simulink model "deadbeat_smm_with_lqr"  (R2015a)
settings: Solver=FixedStepDiscrete  SolverMode=SingleTasking  StartTime=0.0  StopTime=inf  FixedStep=sample_time  RelTol=1e-3
undefined symbols (not defined in the file or in its folder): A_kalman_fourbar_gear, A_kalman_transverse, A_kalman_vertical, A_lpf_accelerometer, A_lpf_fourbar_angles, A_lpf_imu, A_lpf_lateral_angle, B1_lpf_accelerometer, B1_lpf_fourbar_angles, B1_lpf_imu, B1_lpf_lateral_angle, B2_lpf_accelerometer, B2_lpf_fourbar_angles, B2_lpf_imu, B2_lpf_lateral_angle, B_dx_versus_x0, B_kalman_fourbar_gear, B_kalman_transverse, B_kalman_vertical, backwards_K_sag_of_t, backwards_P_sag_of_t, C_kalman_fourbar_gear, C_kalman_transverse, C_kalman_vertical, com_leg_motor, com_torso, contact_threshold, control_start_time, d_ankle_to_foot, d_vertical_com, desired_com_forward_velocity, desired_com_lateral_velocity, desired_initial_leg_roll_left, desired_initial_leg_roll_right, desired_stance_beta2, desired_standing_torso_pitch, desired_standing_torso_roll, desired_standing_z, desired_torso_pitch, desired_torso_roll, Discrete, enable_bouncing, fcut_contact, fdesignblkfcn, forward_dx_of_dxstar, forward_x_of_dxstar, g, gcbh, HIP_MTR_MAX_CONT_TORQUE, HIP_MTR_MAX_TORQUE, i_leg_motor, i_robot, i_torso, initial_dx_estimate, initial_dy_estimate, initial_dz_estimate, initial_leg_selection, initial_z_estimate, k_lateral_accel_for_torso_roll, k_lateral_swing_on_boom ... (+77)
libraries: simulink x21, ctrlSharedLib x7, dsparch4 x3
(part 3 of 5)

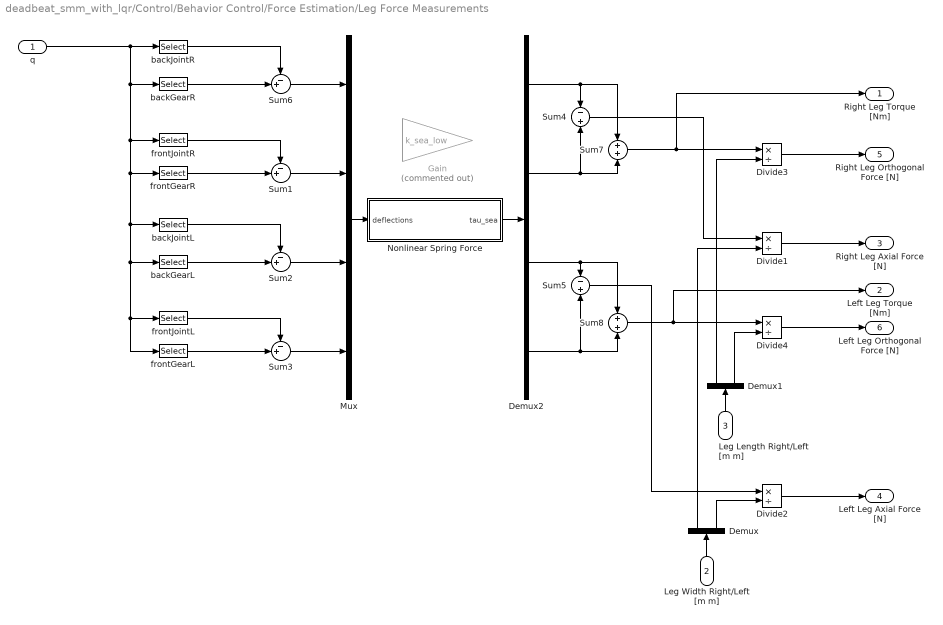
== system deadbeat_smm_with_lqr/Control/Behavior Control/Force Estimation/Leg Force Measurements ==
  q : Inport
  Leg Width Right/Left [m m] : Inport  Port=2
  Leg Length Right/Left [m m] : Inport  Port=3
  Demux : Demux  Outputs=2
  Demux1 : Demux  Outputs=2
  Demux2 : Demux
  Divide{1..4} (4 alike) : Product  Inputs=*/
  Gain : Gain  Commented=on  Gain=k_sea_low
  Mux : Mux
  Nonlinear Spring Force : MATLAB Function  TreatAsAtomicUnit=on
  Sum{1..3,6} (4 alike) : Sum  Inputs=-+|
  Sum4 : Sum  Inputs=-|+
  Sum5 : Sum  Inputs=-|+
  Sum7 : Sum  Inputs=+|+
  Sum8 : Sum  Inputs=+|+
  backGearL : Selector  InputPortWidth=13  Indices=[6]
  backGearR : Selector  InputPortWidth=13  Indices=[2]
  backJointL : Selector  InputPortWidth=13  Indices=[5]
  backJointR : Selector  InputPortWidth=13  Indices=[1]
  frontGearL : Selector  InputPortWidth=13  Indices=[8]
  frontGearR : Selector  InputPortWidth=13  Indices=[4]
  frontJointL : Selector  InputPortWidth=13  Indices=[7]
  frontJointR : Selector  InputPortWidth=13  Indices=[3]
  Right Leg Torque [Nm] : Outport
  Left Leg Torque [Nm] : Outport  Port=2
  Right Leg Axial Force [N] : Outport  Port=3
  Left Leg Axial Force [N] : Outport  Port=4
  Right Leg Orthogonal Force [N] : Outport  Port=5
  Left Leg Orthogonal Force [N] : Outport  Port=6
  wires:
  Nonlinear Spring Force/1(tau_sea) -> Demux2/1
  Mux/1 -> Nonlinear Spring Force/1(deflections)
  Divide4/1 -> Left Leg Orthogonal Force [N]/1
  Divide3/1 -> Right Leg Orthogonal Force [N]/1
  Leg Length Right/Left [m m]/1 -> Demux1/1
  Demux1/2 -> Divide4/2
  Demux1/1 -> Divide3/2
  Sum8/1 -> Left Leg Torque [Nm]/1, Divide4/1
  Sum7/1 -> Right Leg Torque [Nm]/1, Divide3/1
  Demux2/3 -> Sum5/1, Sum8/1
  Divide2/1 -> Left Leg Axial Force [N]/1
  Divide1/1 -> Right Leg Axial Force [N]/1
  Demux/2 -> Divide2/2
  Demux/1 -> Divide1/2
  Leg Width Right/Left [m m]/1 -> Demux/1
  Sum5/1 -> Divide2/1
  Sum4/1 -> Divide1/1
  Demux2/4 -> Sum8/2, Sum5/2
  Demux2/2 -> Sum4/2, Sum7/2
  Demux2/1 -> Sum7/1, Sum4/1
  q/1 -> backJointR/1, frontJointR/1, frontGearR/1, backGearL/1, frontGearL/1, frontJointL/1, backJointL/1, backGearR/1
  backGearR/1 -> Sum6/2
  frontJointR/1 -> Sum1/1
  frontGearR/1 -> Sum1/2
  backJointR/1 -> Sum6/1
  Sum1/1 -> Mux/2
  Sum6/1 -> Mux/1
  backGearL/1 -> Sum2/2
  frontJointL/1 -> Sum3/1
  frontGearL/1 -> Sum3/2
  backJointL/1 -> Sum2/1
  Sum2/1 -> Mux/3
  Sum3/1 -> Mux/4

== system deadbeat_smm_with_lqr/Control/Behavior Control/Force Estimation/Leg Plane GRF ==
  Axial Force [N] : Inport
  Orthogonal Force [N] : Inport  Port=2
  Torso Pitch [rad] : Inport  Port=3
  Leg Angle [rad] : Inport  Port=4
  Gain : Gain  Gain=-1
  Product : Product
  Product1 : Product
  Sum : Sum  Inputs=++|
  Sum1 : Sum  Inputs=+|+
  Trigonometric Function : Trigonometry  Operator=cos
  Trigonometric Function1 : Trigonometry
  Vertical Force [N] : Outport
  wires:
  Gain/1 -> Sum1/1
  Sum/1 -> Trigonometric Function1/1, Trigonometric Function/1
  Product/1 -> Gain/1
  Trigonometric Function/1 -> Product/2
  Torso Pitch [rad]/1 -> Sum/1
  Leg Angle [rad]/1 -> Sum/2
  Axial Force [N]/1 -> Product/1
  Orthogonal Force [N]/1 -> Product1/1
  Trigonometric Function1/1 -> Product1/2
  Sum1/1 -> Vertical Force [N]/1
  Product1/1 -> Sum1/2

== system deadbeat_smm_with_lqr/Control/Behavior Control/Primary and Lateral Behavior/Circular Buffer ==
  Flight [1/0] : Inport
  Exiting Stance [1/0] : Inport  Port=2
  Hopping [1/0] : Inport  Port=3
  dX [m/s] : Inport  Port=4
  dY [m/s] : Inport  Port=5
  X Foot Correction [m] : Inport  Port=6
  Y Foot Correction [m] : Inport  Port=7
  target dX [m/s] : Inport  Port=8
  target dY [m/s] : Inport  Port=9
  Buffer : MATLAB Function  TreatAsAtomicUnit=on  SystemSampleTime=sample_time
  Buffer1 : MATLAB Function  TreatAsAtomicUnit=on  SystemSampleTime=sample_time
  Buffer2 : MATLAB Function  TreatAsAtomicUnit=on  SystemSampleTime=sample_time
  Buffer3 : MATLAB Function  TreatAsAtomicUnit=on  SystemSampleTime=sample_time
  Buffer4 : MATLAB Function  TreatAsAtomicUnit=on  SystemSampleTime=sample_time
  Buffer5 : MATLAB Function  TreatAsAtomicUnit=on  SystemSampleTime=sample_time
  Buffer6 : MATLAB Function  TreatAsAtomicUnit=on  SystemSampleTime=sample_time
  Buffer7 : MATLAB Function  TreatAsAtomicUnit=on  SystemSampleTime=sample_time
  Demux : Demux  Outputs=6
  Detect Decrease : simulink/Logic and Bit Operations/Detect Decrease  vinit=0.0  InputProcessing=Inherited  OutDataTypeStr=boolean
  Enabled on Touchdown : Subsystem  TreatAsAtomicUnit=on
  Logical Operator : Logic  AllPortsSameDT=off  OutDataTypeStr=boolean
  Mux : Mux  Inputs=6
  buffer size5 : Constant  Value=recorded_steps
  "dX Touchdown History " : Outport
  X Foot Correction History : Outport  Port=2
  dX Takeoff History : Outport  Port=3
  "dY Touchdown History " : Outport  Port=4
  Y Foot Correction History : Outport  Port=5
  dY Takeoff History : Outport  Port=6
  target dX History : Outport  Port=7
  target dY History : Outport  Port=8
  wires:
  Buffer/1(buffer) -> "dX Touchdown History "/1
  Detect Decrease/1 -> Enabled on Touchdown/Enable
  Buffer1/1(buffer) -> X Foot Correction History/1
  Buffer2/1(buffer) -> dX Takeoff History/1
  Demux/1 -> Buffer/1(data)
  Demux/3 -> Buffer1/1(data)
  X Foot Correction [m]/1 -> Mux/3
  Buffer3/1(buffer) -> "dY Touchdown History "/1
  Buffer4/1(buffer) -> Y Foot Correction History/1
  Demux/2 -> Buffer3/1(data)
  Buffer5/1(buffer) -> dY Takeoff History/1
  Y Foot Correction [m]/1 -> Mux/4
  Demux/4 -> Buffer4/1(data)
  target dX [m/s]/1 -> Mux/5
  Buffer6/1(buffer) -> target dX History/1
  Buffer7/1(buffer) -> target dY History/1
  buffer size5/1 -> Buffer2/3(buffer_size), Buffer/3(buffer_size), Buffer7/3(buffer_size), Buffer6/3(buffer_size), Buffer4/3(buffer_size), Buffer1/3(buffer_size), Buffer3/3(buffer_size), Buffer5/3(buffer_size)
  Demux/6 -> Buffer7/1(data)
  Demux/5 -> Buffer6/1(data)
  target dY [m/s]/1 -> Mux/6
  Exiting Stance [1/0]/1 -> Buffer/2(trigger), Buffer7/2(trigger), Buffer6/2(trigger), Buffer4/2(trigger), Buffer1/2(trigger), Buffer3/2(trigger), Buffer2/2(trigger), Buffer5/2(trigger)
  Hopping [1/0]/1 -> Logical Operator/1
  dY [m/s]/1 -> Buffer5/1(data), Mux/2
  dX [m/s]/1 -> Buffer2/1(data), Mux/1
  Flight [1/0]/1 -> Logical Operator/2
  Logical Operator/1 -> Detect Decrease/1
  Mux/1 -> Enabled on Touchdown/1(In)
  Enabled on Touchdown/1(Out) -> Demux/1

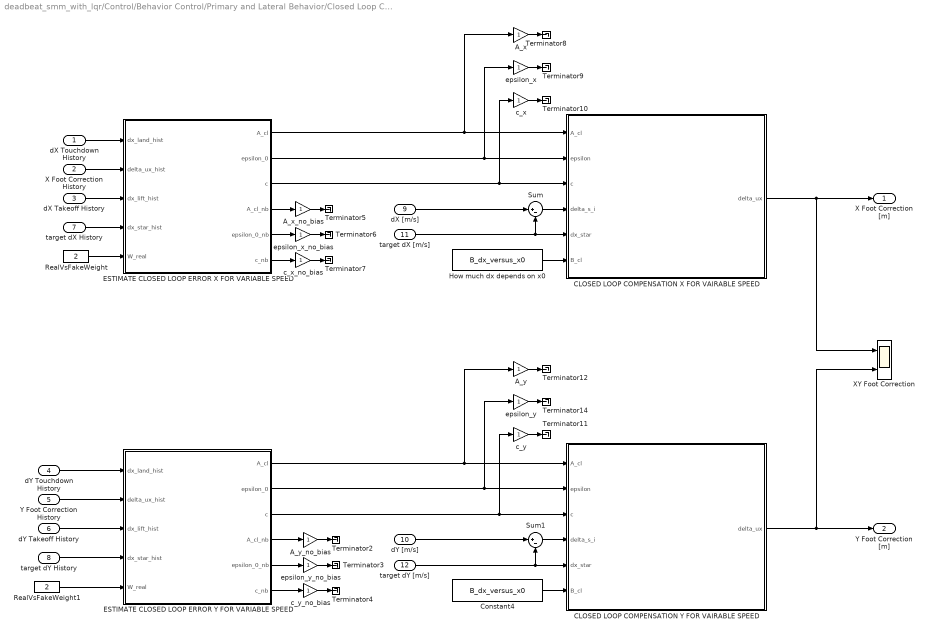
== system deadbeat_smm_with_lqr/Control/Behavior Control/Primary and Lateral Behavior/Closed Loop Compensation ==
  dX Touchdown History : Inport
  X Foot Correction History : Inport  Port=2
  dX Takeoff History : Inport  Port=3
  dY Touchdown History : Inport  Port=4
  Y Foot Correction History : Inport  Port=5
  dY Takeoff History : Inport  Port=6
  target dX History : Inport  Port=7
  target dY History : Inport  Port=8
  dX [m/s] : Inport  Port=9
  dY [m/s] : Inport  Port=10
  target dX [m/s] : Inport  Port=11
  "target dY [m/s] " : Inport  Port=12
  A_x : Gain
  A_x_no_bias : Gain
  A_y : Gain
  A_y_no_bias : Gain
  CLOSED LOOP COMPENSATION X FOR VAIRABLE SPEED : MATLAB Function  TreatAsAtomicUnit=on
  CLOSED LOOP COMPENSATION Y FOR VAIRABLE SPEED : MATLAB Function  TreatAsAtomicUnit=on
  Constant4 : Constant  Value=B_dx_versus_x0
  ESTIMATE CLOSED LOOP ERROR X FOR VARIABLE SPEED : MATLAB Function  TreatAsAtomicUnit=on
  ESTIMATE CLOSED LOOP ERROR Y FOR VARIABLE SPEED : MATLAB Function  TreatAsAtomicUnit=on
  How much dx depends on x0 : Constant  Value=B_dx_versus_x0
  RealVsFakeWeight : Constant  Value=2
  RealVsFakeWeight1 : Constant  Value=2
  Sum : Sum  Inputs=|+-
  Sum1 : Sum  Inputs=|+-
  Terminator{2..12,14} (12 alike) : Terminator
  XY Foot Correction : Scope  NumInputPorts=2
      settings: YMin=-1~-0.8  YMax=1~1.4  SaveName=ScopeData39  SampleInput=on
  c_x : Gain
  c_x_no_bias : Gain
  c_y : Gain
  c_y_no_bias : Gain
  epsilon_x : Gain
  epsilon_x_no_bias : Gain
  epsilon_y : Gain
  epsilon_y_no_bias : Gain
  X Foot Correction [m] : Outport
  Y Foot Correction [m] : Outport  Port=2
  wires:
  c_y/1 -> Terminator11/1
  epsilon_y/1 -> Terminator14/1
  A_y/1 -> Terminator12/1
  ESTIMATE CLOSED LOOP ERROR Y FOR VARIABLE SPEED/1(A_cl) -> CLOSED LOOP COMPENSATION Y FOR VAIRABLE SPEED/1(A_cl), A_y/1
  ESTIMATE CLOSED LOOP ERROR Y FOR VARIABLE SPEED/2(epsilon_0) -> CLOSED LOOP COMPENSATION Y FOR VAIRABLE SPEED/2(epsilon), epsilon_y/1
  ESTIMATE CLOSED LOOP ERROR Y FOR VARIABLE SPEED/3(c) -> CLOSED LOOP COMPENSATION Y FOR VAIRABLE SPEED/3(c), c_y/1
  c_x/1 -> Terminator10/1
  epsilon_x/1 -> Terminator9/1
  A_x/1 -> Terminator8/1
  ESTIMATE CLOSED LOOP ERROR X FOR VARIABLE SPEED/1(A_cl) -> CLOSED LOOP COMPENSATION X FOR VAIRABLE SPEED/1(A_cl), A_x/1
  ESTIMATE CLOSED LOOP ERROR X FOR VARIABLE SPEED/2(epsilon_0) -> CLOSED LOOP COMPENSATION X FOR VAIRABLE SPEED/2(epsilon), epsilon_x/1
  ESTIMATE CLOSED LOOP ERROR X FOR VARIABLE SPEED/3(c) -> CLOSED LOOP COMPENSATION X FOR VAIRABLE SPEED/3(c), c_x/1
  ESTIMATE CLOSED LOOP ERROR Y FOR VARIABLE SPEED/6(c_nb) -> c_y_no_bias/1
  ESTIMATE CLOSED LOOP ERROR Y FOR VARIABLE SPEED/5(epsilon_0_nb) -> epsilon_y_no_bias/1
  ESTIMATE CLOSED LOOP ERROR Y FOR VARIABLE SPEED/4(A_cl_nb) -> A_y_no_bias/1
  c_y_no_bias/1 -> Terminator4/1
  epsilon_y_no_bias/1 -> Terminator3/1
  A_y_no_bias/1 -> Terminator2/1
  c_x_no_bias/1 -> Terminator7/1
  epsilon_x_no_bias/1 -> Terminator6/1
  A_x_no_bias/1 -> Terminator5/1
  ESTIMATE CLOSED LOOP ERROR X FOR VARIABLE SPEED/4(A_cl_nb) -> A_x_no_bias/1
  ESTIMATE CLOSED LOOP ERROR X FOR VARIABLE SPEED/5(epsilon_0_nb) -> epsilon_x_no_bias/1
  ESTIMATE CLOSED LOOP ERROR X FOR VARIABLE SPEED/6(c_nb) -> c_x_no_bias/1
  CLOSED LOOP COMPENSATION Y FOR VAIRABLE SPEED/1(delta_ux) -> Y Foot Correction [m]/1, XY Foot Correction/2
  CLOSED LOOP COMPENSATION X FOR VAIRABLE SPEED/1(delta_ux) -> X Foot Correction [m]/1, XY Foot Correction/1
  Sum1/1 -> CLOSED LOOP COMPENSATION Y FOR VAIRABLE SPEED/4(delta_s_i)
  dY Touchdown History/1 -> ESTIMATE CLOSED LOOP ERROR Y FOR VARIABLE SPEED/1(dx_land_hist)
  dX [m/s]/1 -> Sum/1
  dX Touchdown History/1 -> ESTIMATE CLOSED LOOP ERROR X FOR VARIABLE SPEED/1(dx_land_hist)
  dX Takeoff History/1 -> ESTIMATE CLOSED LOOP ERROR X FOR VARIABLE SPEED/3(dx_lift_hist)
  X Foot Correction History/1 -> ESTIMATE CLOSED LOOP ERROR X FOR VARIABLE SPEED/2(delta_ux_hist)
  target dX History/1 -> ESTIMATE CLOSED LOOP ERROR X FOR VARIABLE SPEED/4(dx_star_hist)
  target dX [m/s]/1 -> CLOSED LOOP COMPENSATION X FOR VAIRABLE SPEED/5(dx_star), Sum/2
  Sum/1 -> CLOSED LOOP COMPENSATION X FOR VAIRABLE SPEED/4(delta_s_i)
  How much dx depends on x0/1 -> CLOSED LOOP COMPENSATION X FOR VAIRABLE SPEED/6(B_cl)
  RealVsFakeWeight/1 -> ESTIMATE CLOSED LOOP ERROR X FOR VARIABLE SPEED/5(W_real)
  dY [m/s]/1 -> Sum1/1
  dY Takeoff History/1 -> ESTIMATE CLOSED LOOP ERROR Y FOR VARIABLE SPEED/3(dx_lift_hist)
  Y Foot Correction History/1 -> ESTIMATE CLOSED LOOP ERROR Y FOR VARIABLE SPEED/2(delta_ux_hist)
  target dY History/1 -> ESTIMATE CLOSED LOOP ERROR Y FOR VARIABLE SPEED/4(dx_star_hist)
  "target dY [m/s] "/1 -> CLOSED LOOP COMPENSATION Y FOR VAIRABLE SPEED/5(dx_star), Sum1/2
  Constant4/1 -> CLOSED LOOP COMPENSATION Y FOR VAIRABLE SPEED/6(B_cl)
  RealVsFakeWeight1/1 -> ESTIMATE CLOSED LOOP ERROR Y FOR VARIABLE SPEED/5(W_real)

== system deadbeat_smm_with_lqr/Control/Behavior Control/Primary and Lateral Behavior/Enabled on Takeoff ==
  In : Inport
  Enable : EnablePort
  Out : Outport
  wires:
  In/1 -> Out/1

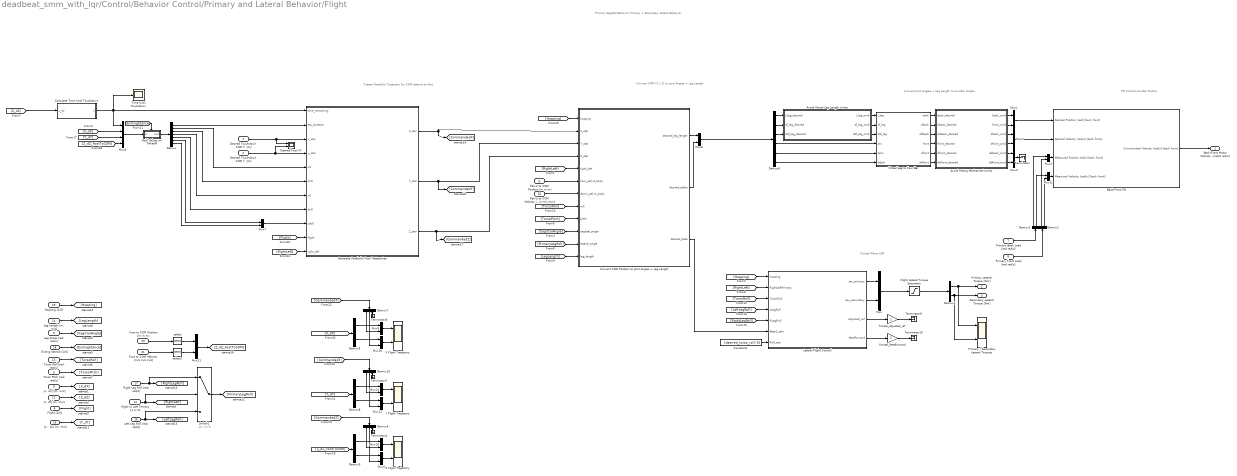
== system deadbeat_smm_with_lqr/Control/Behavior Control/Primary and Lateral Behavior/Flight ==
  note: Frontal Plane LQR
  note: PD Control Fourbar Motors
  note: Convert Joint Angles + Leg Length
      | to Fourbar Angles
  note: Convert COM (X,Y,Z) to
      | Joint Angles + Leg Length
  note: Create Parabolic
      | Trajectory for COM relative to foot
  note: Primary Sagittal Behavior
      | Primary + Secondary Lateral Behavior
  Desired Touchdown COM X  [m] : Inport
  Desired Touchdown COM Y  [m] : Inport  Port=2
  Torso Pitch [rad rad/s] : Inport  Port=3
  Flight [1/0] : Inport  Port=4
  Leg Angle [rad rad/s] : Inport  Port=5
  "[x, dx] [m, m/s]" : Inport  Port=6
  Primary Back Load [rad rad/s] : Inport  Port=7
  Primary Front Load [rad rad/s] : Inport  Port=8
  Pelvis to COM Position [m m m] : Inport  Port=9
  Pelvis to COM Velocity [m/s m/s m/s] : Inport  Port=10
  "[z, dz] [m, m/s]" : Inport  Port=11
  Right or Left Primary [1 or 0] : Inport  Port=12
  Torso Roll [rad rad/s] : Inport  Port=13
  "Leg Length [m, m/s]" : Inport  Port=14
  "[y,  dy] [m, m/s]" : Inport  Port=15
  "Left Leg Roll [rad, rad/s]" : Inport  Port=16
  "Right Leg Roll [rad, rad/s]" : Inport  Port=17
  Exiting Stance [1/0] : Inport  Port=18
  Hopping [1/0] : Inport  Port=19
  Foot to COM Position [m m m] : Inport  Port=20
  Foot to COM Velocity [m/s m/s m/s] : Inport  Port=21
  Avoid Hitting Mechanical Limits : MATLAB Function  TreatAsAtomicUnit=on
  Avoid Virtual Leg Length Limits : MATLAB Function  TreatAsAtomicUnit=on
  Back/Front PD : Subsystem
  Calculate Time Until Touchdown : MATLAB Function  TreatAsAtomicUnit=on
  Constant1 : Constant  Value=[desired_torso_roll; 0]
  "Convert COM Position to Joint Angles + Leg Length " : MATLAB Function  TreatAsAtomicUnit=on
  Demux : Demux  Outputs=7
  Demux{1..3,5,8..9} (6 alike) : Demux  Outputs=2
  Demux10 : Demux  Outputs=3
  Demux4 : Demux  Outputs=3
  Demux6 : Demux  Outputs=6
  Demux7 : Demux  Outputs=3
  Desired Foot XY : Scope  NumInputPorts=2
      settings: YMin=-1~-0.8  YMax=1~1.4  SaveName=ScopeData38  SampleInput=on
  Flight Lateral Torque Saturation : Saturate  UpperLimit=HIP_MTR_MAX_CONT_TORQUE  LowerLimit=-HIP_MTR_MAX_CONT_TORQUE
      settings: AttributesFormatString=Top: %<UpperLimit>\nBottom: %<LowerLimit>
  Generate Parabolic Foot Trajectories : MATLAB Function  TreatAsAtomicUnit=on
  Hold Values on Takeoff : Subsystem
  Lateral Flight Control : MATLAB Function  TreatAsAtomicUnit=on
  Mux{,1..5,7..13,15,21} (15 alike) : Mux  Inputs=2
  Mux6 : Mux
  Primary / Secondary Lateral Torques : Scope  NumInputPorts=2
      settings: YMin=-1~-0.8  YMax=1~1.4  SaveName=ScopeData32  SampleInput=on
  Switch1 : Switch  Criteria=u2 ~= 0
  Terminator{,4,6..7,9..10} (6 alike) : Terminator
  Time Until Touchdown : Scope
      settings: YMin=-1  YMax=1  SaveName=ScopeData37  SampleInput=on
  Virtual Leg to Four Bar : MATLAB Function  TreatAsAtomicUnit=on
  X Flight Trajectory : Scope  NumInputPorts=2
      settings: YMin=-1~-0.8  YMax=1~1.4  SaveName=ScopeData3  SampleInput=on
  Y Flight Trajectory : Scope  NumInputPorts=2
      settings: YMin=-1~-0.8  YMax=1~1.4  SaveName=ScopeData4  SampleInput=on
  Z Flight Trajectory : Scope  NumInputPorts=2
      settings: YMin=-1~-0.8  YMax=1~1.4  SaveName=ScopeData7  SampleInput=on
  frontal_adjusted_ref : Gain
  frontal_feedforward : Gain
  select : Selector  InputPortWidth=3  Indices=[3]
  select1 : Selector  InputPortWidth=3  Indices=[3]
  Back/Front Motor Velocity [rad/s rad/s] : Outport
  Primary Lateral Torque [Nm] : Outport  Port=2
  Secondary Lateral Torque [Nm] : Outport  Port=3
  wires:
  Mux3/1 -> Terminator/1
  Generate Parabolic Foot Trajectories/3(Z_star) -> [CommandedZ], "Convert COM Position to Joint Angles + Leg Length "/4(Z_star)
  [CommandedZ] -> Demux4/1
  [CommandedY] -> Demux10/1
  [CommandedX] -> Demux7/1
  Demux10/3 -> Terminator7/1
  [Y_dY] -> Demux8/1
  Demux10/2 -> Mux12/2
  Demux10/1 -> Mux13/2
  Demux8/2 -> Mux12/1
  Demux8/1 -> Mux13/1
  Mux12/1 -> Y Flight Trajectory/2
  Mux13/1 -> Y Flight Trajectory/1
  Demux7/3 -> Terminator6/1
  [X_dX] -> Demux5/1
  Demux7/2 -> Mux10/2
  Demux7/1 -> Mux9/2
  Demux5/2 -> Mux10/1
  Demux5/1 -> Mux9/1
  Mux10/1 -> X Flight Trajectory/2
  Mux9/1 -> X Flight Trajectory/1
  Demux4/3 -> Terminator4/1
  Demux4/2 -> Mux5/2
  Demux4/1 -> Mux15/2
  Demux9/2 -> Mux5/1
  Demux9/1 -> Mux15/1
  [Z_dZ_FootToCOM] -> Demux9/1
  [Z_dZ_FootToCOM] -> Mux6/4
  Mux5/1 -> Z Flight Trajectory/2
  Mux15/1 -> Z Flight Trajectory/1
  Mux21/1 -> [Z_dZ_FootToCOM]
  select1/1 -> Mux21/2
  select/1 -> Mux21/1
  Foot to COM Velocity [m/s m/s m/s]/1 -> select1/1
  Foot to COM Position [m m m]/1 -> select/1
  Demux/7 -> Mux7/2
  Demux/6 -> Mux7/1
  Demux/5 -> Generate Parabolic Foot Trajectories/8(dy0)
  Demux/4 -> Generate Parabolic Foot Trajectories/7(y0)
  Demux/3 -> Generate Parabolic Foot Trajectories/6(dx0)
  Demux/2 -> Generate Parabolic Foot Trajectories/5(x0)
  [Flight] -> Generate Parabolic Foot Trajectories/10(flight)
  Hopping [1/0]/1 -> [Hopping]
  [Hopping] -> Lateral Flight Control/1(hopping)
  Mux/1 -> Flight Lateral Torque Saturation/1
  [Hopping] -> "Convert COM Position to Joint Angles + Leg Length "/1(hopping)
  frontal_adjusted_ref/1 -> Terminator9/1
  frontal_feedforward/1 -> Terminator10/1
  Flight Lateral Torque Saturation/1 -> Demux1/1
  "Convert COM Position to Joint Angles + Leg Length "/3(desired_beta) -> Lateral Flight Control/6(Beta1_star)
  Demux1/2 -> Secondary Lateral Torque [Nm]/1, Primary / Secondary Lateral Torques/2
  Demux1/1 -> Primary Lateral Torque [Nm]/1, Primary / Secondary Lateral Torques/1
  Exiting Stance [1/0]/1 -> [ExitingStance]
  Switch1/1 -> [PrimaryLegRoll]
  Right or Left Primary [1 or 0]/1 -> [RightLeft], Switch1/2
  "Right Leg Roll [rad, rad/s]"/1 -> [RightLegRoll], Switch1/1
  [RightLegRoll] -> Lateral Flight Control/5(RLegRoll)
  [LeftLegRoll] -> Lateral Flight Control/4(LLegRoll)
  "Left Leg Roll [rad, rad/s]"/1 -> [LeftLegRoll], Switch1/3
  Lateral Flight Control/1(tau_primary) -> Mux/1
  Lateral Flight Control/2(tau_secondary) -> Mux/2
  Lateral Flight Control/4(feedforward) -> frontal_feedforward/1
  Lateral Flight Control/3(adjusted_ref) -> frontal_adjusted_ref/1
  Constant1/1 -> Lateral Flight Control/7(Roll_star)
  [TorsoRoll] -> Lateral Flight Control/3(TorsoRoll)
  [RightLeft] -> Lateral Flight Control/2(RightLeftPrimary)
  Desired Touchdown COM Y  [m]/1 -> Generate Parabolic Foot Trajectories/4(y_star), Desired Foot XY/2
  Demux6/3 -> Avoid Virtual Leg Length Limits/3(ddl_leg_desired)
  Demux6/2 -> Avoid Virtual Leg Length Limits/2(dl_leg_desired)
  Demux6/1 -> Avoid Virtual Leg Length Limits/1(l_leg_desired)
  Avoid Virtual Leg Length Limits/3(ddl_leg_cmd) -> Virtual Leg to Four Bar/3(ddl_leg)
  Avoid Virtual Leg Length Limits/2(dl_leg_cmd) -> Virtual Leg to Four Bar/2(dl_leg)
  Avoid Virtual Leg Length Limits/1(l_leg_cmd) -> Virtual Leg to Four Bar/1(l_leg)
  Calculate Time Until Touchdown/1(t) -> Generate Parabolic Foot Trajectories/1(time_remaining), Time Until Touchdown/1, Mux6/1
  [Z_dZ] -> Calculate Time Until Touchdown/1(z_dz)
  [Y_dY] -> Mux6/3
  "[y,  dy] [m, m/s]"/1 -> [Y_dY]
  Desired Touchdown COM X  [m]/1 -> Generate Parabolic Foot Trajectories/3(x_star), Desired Foot XY/1
  "[z, dz] [m, m/s]"/1 -> [Z_dZ]
  "Leg Length [m, m/s]"/1 -> [LegLength]
  Torso Roll [rad rad/s]/1 -> [TorsoRoll]
  "[x, dx] [m, m/s]"/1 -> [X_dX]
  [ExitingStance] -> Hold Values on Takeoff/Trigger
  Flight [1/0]/1 -> [Flight]
  Pelvis to COM Velocity [m/s m/s m/s]/1 -> "Convert COM Position to Joint Angles + Leg Length "/7(dcom_pelvis_body)
  Pelvis to COM Position [m m m]/1 -> "Convert COM Position to Joint Angles + Leg Length "/6(com_pelvis_body)
  [TorsoRoll] -> "Convert COM Position to Joint Angles + Leg Length "/8(roll)
  [LegLength] -> "Convert COM Position to Joint Angles + Leg Length "/12(leg_length)
  [PrimaryLegRoll] -> "Convert COM Position to Joint Angles + Leg Length "/11(lateral_angle)
  [TorsoPitch] -> "Convert COM Position to Joint Angles + Leg Length "/9(pitch)
  Torso Pitch [rad rad/s]/1 -> [TorsoPitch]
  [SagittalAngle] -> "Convert COM Position to Joint Angles + Leg Length "/10(sagittal_angle)
  Leg Angle [rad rad/s]/1 -> [SagittalAngle]
  Mux8/1 -> Demux6/1
  Demux6/4 -> Virtual Leg to Four Bar/4(phi)
  Demux6/5 -> Virtual Leg to Four Bar/5(dphi)
  Demux6/6 -> Virtual Leg to Four Bar/6(ddphi)
  "Convert COM Position to Joint Angles + Leg Length "/1(desired_leg_length) -> Mux8/1
  "Convert COM Position to Joint Angles + Leg Length "/2(desired_alpha) -> Mux8/2
  [RightLeft] -> "Convert COM Position to Joint Angles + Leg Length "/5(right_left)
  Generate Parabolic Foot Trajectories/2(Y_star) -> [CommandedY], "Convert COM Position to Joint Angles + Leg Length "/3(Y_star)
  Generate Parabolic Foot Trajectories/1(X_star) -> "Convert COM Position to Joint Angles + Leg Length "/2(X_star), [CommandedX]
  [X_dX] -> Mux6/2
  Hold Values on Takeoff/1(out) -> Demux/1
  Mux6/1 -> Hold Values on Takeoff/1(in)
  Mux7/1 -> Generate Parabolic Foot Trajectories/9(zdz0)
  Demux/1 -> Generate Parabolic Foot Trajectories/2(est_duration)
  Primary Front Load [rad rad/s]/1 -> Demux2/1
  Primary Back Load [rad rad/s]/1 -> Demux3/1
  Back/Front PD/1(Commanded Velocity [rad/s] [back front]) -> Back/Front Motor Velocity [rad/s rad/s]/1
  Mux2/1 -> Back/Front PD/2(Desired Velocity [rad/s] [back front])
  Avoid Hitting Mechanical Limits/6(ddfront_cmd) -> Mux3/2
  Avoid Hitting Mechanical Limits/5(ddback_cmd) -> Mux3/1
  Avoid Hitting Mechanical Limits/4(dfront_cmd) -> Mux2/2
  Avoid Hitting Mechanical Limits/3(dback_cmd) -> Mux2/1
  Demux2/1 -> Mux4/2
  Avoid Hitting Mechanical Limits/1(back_cmd) -> Mux1/1
  Avoid Hitting Mechanical Limits/2(front_cmd) -> Mux1/2
  Demux3/1 -> Mux4/1
  Demux3/2 -> Mux11/1
  Mux1/1 -> Back/Front PD/1(Desired Position [rad] [back front])
  Mux4/1 -> Back/Front PD/3(Measured Position [rad] [back front])
  Demux2/2 -> Mux11/2
  Mux11/1 -> Back/Front PD/4(Measured Velocity [rad/s] [back front])
  Virtual Leg to Four Bar/6(ddfront) -> Avoid Hitting Mechanical Limits/6(ddfront_desired)
  Virtual Leg to Four Bar/5(dfront) -> Avoid Hitting Mechanical Limits/5(dfront_desired)
  Virtual Leg to Four Bar/4(front) -> Avoid Hitting Mechanical Limits/4(front_desired)
  Virtual Leg to Four Bar/3(ddback) -> Avoid Hitting Mechanical Limits/3(ddback_desired)
  Virtual Leg to Four Bar/2(dback) -> Avoid Hitting Mechanical Limits/2(dback_desired)
  Virtual Leg to Four Bar/1(back) -> Avoid Hitting Mechanical Limits/1(back_desired)
  [RightLeft] -> Generate Parabolic Foot Trajectories/11(right_left)

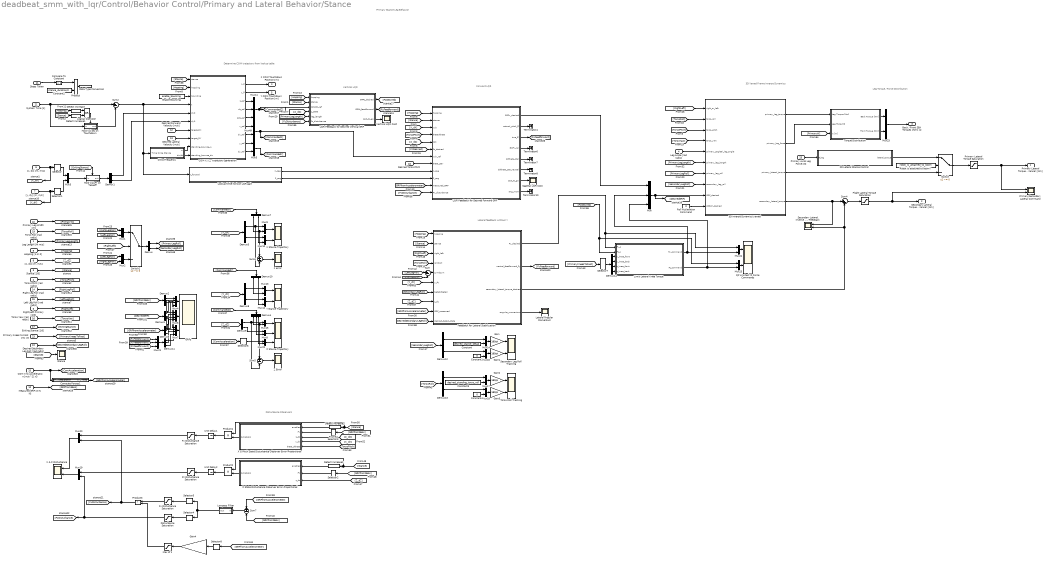
== system deadbeat_smm_with_lqr/Control/Behavior Control/Primary and Lateral Behavior/Stance ==
  note: Leg Torque / Force
      | Distribution
  note: Disturbance Observers
  note: Primary Stance Leg Behavior
  note: Determine COM trajectory
      | from lookup table
  note: Vertical LQR
  note: Forward LQR
  note: 3D Yawed Frame Inverse Dynamics
  note: Lateral feedback without Y
  Leg Length [m m/s] : Inport
  Torso Pitch [rad rad/s] : Inport  Port=2
  Stance [1/0] : Inport  Port=3
  Leg Angle [rad rad/s] : Inport  Port=4
  Right/Left Primary [1/0] : Inport  Port=5
  "[x, dx] [m, m/s]" : Inport  Port=6
  "[y, dy] [m, m/s]" : Inport  Port=7
  "[z, dz] [m, m/s]" : Inport  Port=8
  Hopping [1 or 0] : Inport  Port=9
  Measured GRF [N N N] : Inport  Port=10
  Steps Taken : Inport  Port=11
  Desired Forward Velocity [m/s] : Inport  Port=12
  Desired Lateral Velocity [m/s] : Inport  Port=13
  Right Leg Roll [rad rad/s] : Inport  Port=14
  Left Leg Roll [rad rad/s] : Inport  Port=15
  Torso Yaw [rad rad/s] : Inport  Port=16
  Exiting Stance [1/0] : Inport  Port=17
  Desired Torso Pitch : Inport  Port=18
  Torso Roll [rad rad/s] : Inport  Port=19
  COM XYZ Acceleration [m/s^2] x3 : Inport  Port=20
  System Time [s] : Inport  Port=21
  Primary Leg Width [m] : Inport  Port=22
  Primary Knees to Foot [m] x6 : Inport  Port=23
  Desired Secondary Leg Roll [rad rad/s] : Inport  Port=24
  Primary Axial Leg Force [N] : Inport  Port=25
  2D Lateral Stance Control : MATLAB Function  TreatAsAtomicUnit=on
  3D Inverse Dynamics yawed : MATLAB Function  TreatAsAtomicUnit=on
  COM X,Y,Z  trajectory generation : MATLAB Function  TreatAsAtomicUnit=on
  Chirp Frequency : Subsystem
  Compare To Constant : simulink/Logic and Bit Operations/Compare To Constant  relop=<  const=1  OutDataTypeStr=uint8
  Compute Forces1 : Subsystem
  Constant : Constant  Value=desired_stance_beta2
  Constant1 : Constant  Value=0
  Constant2 : Constant  Value=stance_duration/2
  Constant3 : Constant  Value=desired_standing_torso_roll
  Constant4 : Constant  Value=0
  Data Type Conversion : DataTypeConversion  OutDataTypeStr=double
  Demux{,1,5,7..10,12..13} (9 alike) : Demux  Outputs=2
  Demux{2..4,6,11} (5 alike) : Demux  Outputs=3
  Demux14 : Demux
  Detect Increase{,1..3} (4 alike) : simulink/Logic and Bit Operations/Detect Increase  vinit=0.0  InputProcessing=Inherited  OutDataTypeStr=boolean
  "Disturbance Saturation " : Saturate  UpperLimit=100  LowerLimit=-100
      settings: AttributesFormatString=Top: %<UpperLimit>\nBottom: %<LowerLimit>
  Enable Bouncing : Constant  Value=enable_bouncing  SampleTime=sample_time
  Feedback for Lateral Stabilization : MATLAB Function  TreatAsAtomicUnit=on
  Flight Lateral Torque Saturation : Saturate  UpperLimit=HIP_MTR_MAX_CONT_TORQUE  LowerLimit=-HIP_MTR_MAX_CONT_TORQUE
      settings: AttributesFormatString=Top: %<UpperLimit>\nBottom: %<LowerLimit>
  Fx Disturbance Saturation : Saturate  UpperLimit=100  LowerLimit=-100
      settings: AttributesFormatString=Top: %<UpperLimit>\nBottom: %<LowerLimit>
  "Fx Disturbance Saturation " : Saturate  UpperLimit=100  LowerLimit=-100
      settings: AttributesFormatString=Top: %<UpperLimit>\nBottom: %<LowerLimit>
  Fz Disturbance Saturation : Saturate  UpperLimit=100  LowerLimit=-100
      settings: AttributesFormatString=Top: %<UpperLimit>\nBottom: %<LowerLimit>
  GRFs : Scope  NumInputPorts=3
      settings: TimeRange=37.999  YMin=-1250~-2000~-1250  YMax=1500~3750~1750  SampleInput=on
  Gain{,1..3} (4 alike) : Gain  Gain=180/pi
  Gain4 : Gain  Gain=2/(m_total_real*g)
  Hold Values on Takeoff : Subsystem
  Hold Values on Touchdown : Subsystem
  LQR Feedback for Desired Forward GRF : MATLAB Function  TreatAsAtomicUnit=on
  LQR Feedback for Desired Vertical GRF : MATLAB Function  TreatAsAtomicUnit=on
  Lateral Angular Momentum : Scope
      settings: YMin=-3.5  YMax=4  SaveName=ScopeData20  SampleInput=on
  Limit Lateral Knee Torque : MATLAB Function  TreatAsAtomicUnit=on
  Logical Operator : Logic  Operator=OR  AllPortsSameDT=off  OutDataTypeStr=boolean
  Lookup finite horizon LQR gain : MATLAB Function  TreatAsAtomicUnit=on
  Lowpass Filter : Subsystem  DialogController=fdesignblkfcn  InitFcn=fdesignblkfcn(gcbh, {'InitFcn'});  mask(Lowpass Filter){}
      mask help: Design a lowpass filter
      settings: CopyFcn=fdesignblkfcn(gcbh, {'CopyFcn'});
      mask Help: helpview(mapfilelocation('dsp'), 'dsplowpassfilter');
      mask Display: disp('Lowpass')
  Max of 1 : Saturate  UpperLimit=1  LowerLimit=0
      settings: AttributesFormatString=Top: %<UpperLimit>\nBottom: %<LowerLimit>
  Mux : Mux  Inputs=3
  Mux{1..3,5,8..10,12..20,22..25,49} (21 alike) : Mux  Inputs=2
  Mux11 : Mux  Inputs=3
  Mux21 : Mux  Inputs=3
  Mux4 : Mux
  Mux6 : Mux
  Mux7 : Mux
  Primary Lateral Torque Saturation : Saturate  UpperLimit=max_primary_lateral_stance_torque  LowerLimit=-max_primary_lateral_stance_torque
      settings: AttributesFormatString=Top: %<UpperLimit>\nBottom: %<LowerLimit>
  Primary/Secondary Lateral Command : Scope  NumInputPorts=2
      settings: YMin=40~-5  YMax=150~5  SaveName=ScopeData25  SampleInput=on
  Product{,1..3} (4 alike) : Product
  QP Limited YZ Force Commands : Scope  NumInputPorts=2
      settings: YMin=40~-5  YMax=150~5  SaveName=ScopeData26  SampleInput=on
  Robot is attached to boom? : Constant  Value=robot_is_attached_to_boom
  Roll Accleration Command : Constant  Value=0
  Sagittal LQR Cost : Scope
      settings: YMin=22.5  YMax=62.5  SaveName=ScopeData10  SampleInput=on
  Secondary Lateral Inverse Dynamics / Feedback : Scope  NumInputPorts=2
      settings: YMin=-3.5~-5  YMax=4~5  SaveName=ScopeData9  SampleInput=on
  Secondary Leg Roll Tracking : Scope  NumInputPorts=2
      settings: YMin=-3.5~-5  YMax=4~5  SaveName=ScopeData12  SampleInput=on
  Selector : Selector  InputPortWidth=2  Indices=[2]
  Selector1 : Selector  InputPortWidth=2  Indices=[2]
  Selector{2,4,6,8} (4 alike) : Selector  InputPortWidth=3  Indices=[3]
  Selector3 : Selector  InputPortWidth=3  Indices=[1]
  Selector5 : Selector  InputPortWidth=3  Indices=[1]
  Selector7 : Selector  InputPortWidth=6  Indices=[2 5 3 6]
  Stance : Scope
      settings: YMin=-0.05  YMax=0.11  SaveName=stance_time_history  SampleInput=on
  Sum : Sum  Inputs=|+-
  Sum2 : Sum  Inputs=|+-
  Sum4 : Sum  Inputs=|++
  Sum5 : Sum  Inputs=+-
  Sum6 : Sum  Inputs=+-
  Sum7 : Sum  Inputs=+-
  Switch : Switch  Criteria=u2 ~= 0
  Switch1 : Switch  Criteria=u2 ~= 0
  Terminator{4,6..8,10} (5 alike) : Terminator
  Torque Distribution : Subsystem
  Torso Roll Tracking : Scope  NumInputPorts=2
      settings: YMin=-3.5~-5  YMax=4~5  SaveName=ScopeData15  SampleInput=on
  Unit Delay1 : UnitDelay  SampleTime=sample_time
  Unit Delay2 : UnitDelay  SampleTime=sample_time
  Vertical LQR Cost : Scope
      settings: YMin=11  YMax=16  SaveName=ScopeData18  SampleInput=on
  X & Pitch State Disturbance Observer Error-Proportional : MATLAB Function  TreatAsAtomicUnit=on
  X & Z Disturbance : Scope  NumInputPorts=2
      settings: YMin=-125~-800  YMax=175~700  SaveName=ScopeData16  SampleInput=on
  X Stance Trajectory : Scope  NumInputPorts=2
      settings: YMin=0~-0.02  YMax=0.005~0.03  SaveName=ScopeData8  SampleInput=on
  X error : Scope
      settings: YMin=-0.05  YMax=0.11  SaveName=ScopeData24  SampleInput=on
  Y Stance Trajectory : Scope  NumInputPorts=2
      settings: YMin=0.005~-0.5  YMax=0.1~0.3  SaveName=ScopeData5  SampleInput=on
  Z Error : Scope
      settings: YMin=-0.007  YMax=0.0005  SaveName=ScopeData23  SampleInput=on
  Z Stance Trajectory : Scope  NumInputPorts=3
      settings: YMin=0.85~-0.4~-3  YMax=0.98~0.6~11  SaveName=z_stance_trajectory  SampleInput=on
  Z State Disturbance Observer Error-Proportional : MATLAB Function  TreatAsAtomicUnit=on
  Primary Lateral Torque Command (stance) [Nm] : Outport
  Secondary Lateral Torque Command (stance) [Nm] : Outport  Port=2
  Back / Front SEA Torques [Nm] x2 : Outport  Port=3
  X COM Touchdown Position [m] : Outport  Port=4
  Y COM Touchdown Position [m] : Outport  Port=5
  wires:
  Limit Lateral Knee Torque/1(Fy_command) -> Mux/2, Mux24/2
  Mux25/1 -> QP Limited YZ Force Commands/2
  Mux24/1 -> QP Limited YZ Force Commands/1
  Selector7/1 -> Demux14/1
  Demux14/4 -> Limit Lateral Knee Torque/6(z_knee_back)
  Demux14/3 -> Limit Lateral Knee Torque/5(z_knee_front)
  Demux14/2 -> Limit Lateral Knee Torque/4(y_knee_back)
  Demux14/1 -> Limit Lateral Knee Torque/3(y_knee_front)
  [PrimaryKneesToFoot] -> Selector7/1
  Primary Knees to Foot [m] x6/1 -> [PrimaryKneesToFoot]
  Feedback for Lateral Stabilization/2(neutral_feedforward_Fy) -> [FyFeedforward]
  LQR Feedback for Desired Forward GRF/2(netural_pitch_ff) -> Terminator4/1
  LQR Feedback for Desired Forward GRF/3(true_ff) -> [FxFeedforward]
  Compute Forces1/1(XYZ Force) -> [GRFfromAccelerometer]
  [FyFeedforward] -> Mux21/2
  [Z_dZ] -> Feedback for Lateral Stabilization/8(z_dz)
  [FzDesired] -> Mux25/1, Limit Lateral Knee Torque/2(Fz_s)
  [FzDesired] -> LQR Feedback for Desired Forward GRF/6(Fz_desired)
  [FxFeedforward] -> Mux21/1
  Mux23/1 -> Back / Front SEA Torques [Nm] x2/1
  Torque Distribution/2(Front Torque [Nm]) -> Mux23/2
  Torque Distribution/1(Back Torque [Nm]) -> Mux23/1
  Primary Leg Width [m]/1 -> [PrimaryW]
  3D Inverse Dynamics yawed/2(primary_leg_force) -> Torque Distribution/2(Leg Force [N])
  [PrimaryW] -> Torque Distribution/3(w [m])
  3D Inverse Dynamics yawed/1(primary_leg_torque) -> Torque Distribution/1(Leg Torque [Nm])
  Selector6/1 -> Mux22/1
  [ComAcceleration] -> Selector6/1
  Mux22/1 -> Z Stance Trajectory/3
  Sum5/1 -> Z Error/1
  [CommandedZ] -> Demux4/1
  Demux4/3 -> Mux22/2
  Demux4/2 -> Mux8/2
  Demux4/1 -> Sum5/1, Mux15/2
  Demux9/2 -> Mux8/1
  Demux9/1 -> Sum5/2, Mux15/1
  [Z_dZ] -> Demux9/1
  Mux8/1 -> Z Stance Trajectory/2
  Mux15/1 -> Z Stance Trajectory/1
  [FzFeedforward] -> Mux21/3
  Mux21/1 -> Demux11/1
  LQR Feedback for Desired Vertical GRF/2(GRFz_feedforward) -> [FzFeedforward]
  [GRFfromAccelerometer] -> Demux6/1
  COM XYZ Acceleration [m/s^2] x3/1 -> [ComAcceleration], Compute Forces1/1(XYZ Acceleration)
  Selector4/1 -> "Disturbance Saturation "/1
  [GRFfromSEAs] -> Sum7/2
  Mux19/1 -> X & Z Disturbance/2
  [Stance] -> Detect Increase2/1, Product2/1
  Z State Disturbance Observer Error-Proportional/1(d_hat_tp1) -> Product2/2
  [Stance] -> Detect Increase3/1, Product1/1
  X & Pitch State Disturbance Observer Error-Proportional/1(d_hat_tp1) -> Product1/2
  Product2/1 -> Unit Delay2/1
  Product1/1 -> Unit Delay1/1
  [Z_dZ] -> Z State Disturbance Observer Error-Proportional/3(z_dz)
  [GRFfromSEAs] -> Selector2/1
  Detect Increase2/1 -> Z State Disturbance Observer Error-Proportional/1(enabled)
  Detect Increase3/1 -> X & Pitch State Disturbance Observer Error-Proportional/1(enabled)
  [GRFfromSEAs] -> Selector3/1
  [X_dX] -> X & Pitch State Disturbance Observer Error-Proportional/4(x_dx)
  [TorsoPitch] -> X & Pitch State Disturbance Observer Error-Proportional/5(theta_dtheta)
  [Z_dZ] -> X & Pitch State Disturbance Observer Error-Proportional/3(z_dz)
  "[z, dz] [m, m/s]"/1 -> [Z_dZ]
  Flight Lateral Torque Saturation/1 -> Secondary Lateral Torque Command (stance) [Nm]/1, Primary/Secondary Lateral Command/2
  Demux6/3 -> Mux7/3
  Demux6/2 -> Mux6/3
  Demux6/1 -> Mux4/3
  Feedback for Lateral Stabilization/4(angular_momentum) -> Lateral Angular Momentum/1
  LQR Feedback for Desired Forward GRF/4(GRFx_lqr) -> Terminator6/1
  [Stance] -> COM X,Y,Z  trajectory generation/1(stance)
  Lookup finite horizon LQR gain/2(P_sag) -> LQR Feedback for Desired Forward GRF/10(P_sag)
  [Z_dZ] -> LQR Feedback for Desired Vertical GRF/4(z_state)
  COM X,Y,Z  trajectory generation/3(z_ref) -> Mux11/1
  [Stance] -> LQR Feedback for Desired Forward GRF/2(stance)
  COM X,Y,Z  trajectory generation/6(x_ref) -> Mux49/1
  COM X,Y,Z  trajectory generation/7(dx_ref) -> Mux49/2
  COM X,Y,Z  trajectory generation/8(y_ref) -> Mux5/1
  COM X,Y,Z  trajectory generation/9(dy_ref) -> Mux5/2
  COM X,Y,Z  trajectory generation/1(x_0) -> X COM Touchdown Position [m]/1
  COM X,Y,Z  trajectory generation/4(dz_ref) -> Mux11/2
  COM X,Y,Z  trajectory generation/5(ddz_ref) -> Mux11/3
  Mux11/1 -> [CommandedZ], LQR Feedback for Desired Vertical GRF/3(zdzddz_ref)
  [X_dX] -> LQR Feedback for Desired Forward GRF/3(xdx)
  [TorsoPitch] -> LQR Feedback for Desired Forward GRF/4(thetadtheta)
  Mux49/1 -> [CommandedX], LQR Feedback for Desired Forward GRF/7(xdx_ref)
  Desired Torso Pitch/1 -> LQR Feedback for Desired Forward GRF/8(theta_star)
  Lookup finite horizon LQR gain/1(K_sag) -> LQR Feedback for Desired Forward GRF/9(K_sag)
  [Z_dZ] -> LQR Feedback for Desired Forward GRF/5(zdz)
  Desired Forward Velocity [m/s]/1 -> COM X,Y,Z  trajectory generation/7(target_DX)
  Sum2/1 -> COM X,Y,Z  trajectory generation/4(t), Lookup finite horizon LQR gain/1(t_forward), Chirp Frequency/1(Time Since Stance)
  LQR Feedback for Desired Vertical GRF/1(GRFz_desired) -> [FzDesired]
  Hold Values on Touchdown/1(out) -> Sum2/2
  Stance [1/0]/1 -> [Stance]
  [Stance] -> LQR Feedback for Desired Vertical GRF/2(stance)
  Logical Operator/1 -> Hold Values on Touchdown/Trigger
  "[x, dx] [m, m/s]"/1 -> [X_dX], Selector/1
  Demux1/2 -> COM X,Y,Z  trajectory generation/6(dy0)
  LQR Feedback for Desired Vertical GRF/3(cost_to_go) -> Vertical LQR Cost/1
  LQR Feedback for Desired Forward GRF/5(ddtheta_star) -> Terminator7/1
  LQR Feedback for Desired Forward GRF/6(ddtheta_star_neutral) -> Terminator8/1
  LQR Feedback for Desired Forward GRF/7(cost_to_go) -> Sagittal LQR Cost/1
  LQR Feedback for Desired Forward GRF/8(ang_mom) -> Terminator10/1
  Torso Pitch [rad rad/s]/1 -> [TorsoPitch]
  [RightLeft] -> 3D Inverse Dynamics yawed/1(right_or_left)
  Hopping [1 or 0]/1 -> [Hopping]
  [Hopping] -> COM X,Y,Z  trajectory generation/2(hopping)
  [Hopping] -> LQR Feedback for Desired Forward GRF/1(hopping)
  Measured GRF [N N N]/1 -> [GRFfromSEAs]
  [GRFfromAccelerometer] -> LQR Feedback for Desired Forward GRF/11(measured_GRF)
  Steps Taken/1 -> Compare To Constant/1
  Product/1 -> Data Type Conversion/1
  Constant2/1 -> Product/2
  Detect Increase/1 -> Logical Operator/1
  Detect Increase1/1 -> Logical Operator/2
  Compare To Constant/1 -> Product/1
  [Hopping] -> Detect Increase/1
  [Stance] -> Detect Increase1/1
  Demux1/1 -> COM X,Y,Z  trajectory generation/5(dx0)
  Selector/1 -> Mux3/1
  [Hopping] -> LQR Feedback for Desired Vertical GRF/1(hopping)
  [Stance] -> Feedback for Lateral Stabilization/2(stance)
  [TorsoRoll] -> Feedback for Lateral Stabilization/4(rolldroll)
  COM X,Y,Z  trajectory generation/2(y_0) -> Y COM Touchdown Position [m]/1
  Mux5/1 -> [CommandedY]
  [TorsoPitch] -> 3D Inverse Dynamics yawed/3(torso_pitch)
  [TorsoRoll] -> 3D Inverse Dynamics yawed/2(torso_roll)
  [TorsoYaw] -> 3D Inverse Dynamics yawed/4(torso_yaw)
  [PrimaryLegLength] -> 3D Inverse Dynamics yawed/6(primary_leg_length)
  Leg Angle [rad rad/s]/1 -> 3D Inverse Dynamics yawed/5(primary_sagittal_leg_angle)
  [SecondaryLegRoll] -> 3D Inverse Dynamics yawed/8(secondary_leg_roll)
  [PrimaryLegRoll] -> 3D Inverse Dynamics yawed/7(primary_leg_roll)
  Switch1/1 -> Demux/1
  Demux/2 -> [SecondaryLegRoll]
  Demux/1 -> [PrimaryLegRoll]
  Mux1/1 -> Switch1/1
  Mux2/1 -> Switch1/3
  Right Leg Roll [rad rad/s]/1 -> [RightLegRoll]
  [RightLegRoll] -> Mux1/1
  [LeftLegRoll] -> Mux1/2
  [LeftLegRoll] -> Mux2/1
  [RightLegRoll] -> Mux2/2
  [RightLeft] -> Switch1/2
  "[y, dy] [m, m/s]"/1 -> [Y_dY], Selector1/1
  Mux3/1 -> Hold Values on Takeoff/1(in)
  Hold Values on Takeoff/1(out) -> Demux1/1
  Selector1/1 -> Mux3/2
  Desired Lateral Velocity [m/s]/1 -> COM X,Y,Z  trajectory generation/8(target_DY)
  Torso Yaw [rad rad/s]/1 -> [TorsoYaw]
  Exiting Stance [1/0]/1 -> [ExitingStance]
  [ExitingStance] -> Hold Values on Takeoff/Trigger
  [Hopping] -> Feedback for Lateral Stabilization/1(hopping)
  [GRFfromAccelerometer] -> Feedback for Lateral Stabilization/9(GRF_measured)
  System Time [s]/1 -> Hold Values on Touchdown/1(in), Sum2/1
  Leg Length [m m/s]/1 -> [PrimaryLegLength]
  [PrimaryLegLength] -> LQR Feedback for Desired Vertical GRF/5(leg_length)
  Torso Roll [rad rad/s]/1 -> [TorsoRoll]
  [GRFfromSEAs] -> Demux2/1
  [DesiredGRF] -> Demux3/1
  Mux4/1 -> GRFs/1
  Demux2/1 -> Mux4/1
  Mux6/1 -> GRFs/2
  Mux7/1 -> GRFs/3
  Demux2/2 -> Mux6/1
  Demux2/3 -> Mux7/1
  Demux3/1 -> Mux4/2
  Demux3/2 -> Mux6/2
  Demux3/3 -> Mux7/2
  Mux9/1 -> X Stance Trajectory/1
  Mux10/1 -> X Stance Trajectory/2
  Demux5/2 -> Mux10/1
  Demux7/2 -> Mux10/2
  [X_dX] -> Demux5/1
  Mux13/1 -> Y Stance Trajectory/1
  Mux12/1 -> Y Stance Trajectory/2
  Demux8/1 -> Mux13/1
  Demux8/2 -> Mux12/1
  Demux10/1 -> Mux13/2
  Demux10/2 -> Mux12/2
  [Y_dY] -> Demux8/1
  [CommandedX] -> Demux7/1
  [CommandedY] -> Demux10/1
  Right/Left Primary [1/0]/1 -> [RightLeft]
  Left Leg Roll [rad rad/s]/1 -> [LeftLegRoll]
  LQR Feedback for Desired Forward GRF/1(GRFx_desired) -> Mux/1
  Mux/1 -> 3D Inverse Dynamics yawed/9(GRF_desired), [DesiredGRF]
  Demux11/1 -> Mux4/4
  Demux11/2 -> Mux6/4
  Demux11/3 -> Mux7/4
  Primary Lateral Torque Saturation/1 -> Primary Lateral Torque Command (stance) [Nm]/1, Primary/Secondary Lateral Command/1
  Feedback for Lateral Stabilization/1(Fy_desired) -> Mux24/1, Limit Lateral Knee Torque/1(Fy_s)
  Roll Accleration Command/1 -> 3D Inverse Dynamics yawed/10(ddRoll_desired)
  [LeftLegRoll] -> Sum/1
  [RightLegRoll] -> Sum/2
  [Y_dY] -> Feedback for Lateral Stabilization/6(y_dy)
  [SecondaryLegRoll] -> Feedback for Lateral Stabilization/7(beta2dbeta2)
  Sum/1 -> Feedback for Lateral Stabilization/5(symdsym)
  3D Inverse Dynamics yawed/4(secondary_lateral_torque) -> Sum4/1, Secondary Lateral Inverse Dynamics / Feedback/1
  Switch/1 -> Primary Lateral Torque Saturation/1
  Sum4/1 -> Flight Lateral Torque Saturation/1
  Feedback for Lateral Stabilization/3(secondary_lateral_torque_desired) -> Secondary Lateral Inverse Dynamics / Feedback/2, Sum4/2
  [SecondaryLegRoll] -> Demux12/1
  Mux14/1 -> Gain/1
  Demux12/1 -> Mux14/1
  Constant/1 -> Mux14/2
  Gain/1 -> Secondary Leg Roll Tracking/1
  Gain1/1 -> Secondary Leg Roll Tracking/2
  Mux16/1 -> Gain1/1
  Demux12/2 -> Mux16/1
  Constant1/1 -> Mux16/2
  [TorsoRoll] -> Demux13/1
  Gain2/1 -> Torso Roll Tracking/1
  Gain3/1 -> Torso Roll Tracking/2
  Mux17/1 -> Gain2/1
  Demux13/1 -> Mux17/1
  Constant3/1 -> Mux17/2
  Demux13/2 -> Mux18/1
  Mux18/1 -> Gain3/1
  Constant4/1 -> Mux18/2
  [RightLeft] -> Feedback for Lateral Stabilization/3(right_left)
  Enable Bouncing/1 -> COM X,Y,Z  trajectory generation/3(bouncing)
  Fx Disturbance Saturation/1 -> Mux20/1
  Selector3/1 -> X & Pitch State Disturbance Observer Error-Proportional/2(Fx)
  Unit Delay1/1 -> Fx Disturbance Saturation/1
  Unit Delay2/1 -> Fz Disturbance Saturation/1
  Demux5/1 -> Sum6/2, Mux9/1
  Demux7/1 -> Sum6/1, Mux9/2
  Sum6/1 -> X error/1
  [GRFfromAccelerometer] -> Sum7/1
  Mux20/1 -> X & Z Disturbance/1
  Product3/1 -> [FxDisturbance], Mux20/2
  Sum7/1 -> Lowpass Filter/1(In)
  Selector2/1 -> Z State Disturbance Observer Error-Proportional/2(Fz)
  Chirp Frequency/1(w) -> COM X,Y,Z  trajectory generation/9(standing_bounce_w)
  [Stance] -> Stance/1
  Chirp Frequency/2(dw/dt) -> COM X,Y,Z  trajectory generation/10(standing_bounce_dw)
  Lowpass Filter/1(Out) -> Selector4/1, Selector5/1
  [FxDisturbance] -> LQR Feedback for Desired Forward GRF/12(Fx_disturbance)
  [FzDisturbance] -> LQR Feedback for Desired Vertical GRF/6(Fz_disturbance)
  Limit Lateral Knee Torque/2(Fz_command) -> Mux25/2, Mux/3
  [GRFfromAccelerometer] -> Selector8/1
  Selector8/1 -> Gain4/1
  Gain4/1 -> Max of 1/1
  "Fx Disturbance Saturation "/1 -> Product3/1
  Max of 1/1 -> Product3/2
  "Disturbance Saturation "/1 -> Mux19/2, [FzDisturbance]
  Selector5/1 -> "Fx Disturbance Saturation "/1
  Fz Disturbance Saturation/1 -> Mux19/1
  [DesiredSecondaryLegRoll] -> Feedback for Lateral Stabilization/10(desired_beta2_state)
  Desired Secondary Leg Roll [rad rad/s]/1 -> [DesiredSecondaryLegRoll]
  Primary Axial Leg Force [N]/1 -> 2D Lateral Stance Control/1(F_leg)
  2D Lateral Stance Control/1(lateral_torque) -> Switch/1
  Robot is attached to boom?/1 -> Switch/2
  3D Inverse Dynamics yawed/3(primary_lateral_torque) -> Switch/3
